simulink model "numerical_lagrangian"  (R2024b)
settings: Solver=ode4  StartTime=0.0  StopTime=8  FixedStep=0.001  RelTol=1e-3
InitFcn:
  | run('assignment_block2.m')
values from neighbouring files (symbols this model uses):
  Acoeffs = computeCoefficients(number_coefficients, tA, tB, qa, qdot_a, qddot_a, qb, qdot_b, qddot_b)    [assignment_block2.m]
  Bcoeffs = computeCoefficients(number_coefficients, tA, tB, qa, qdot_a, qddot_a, qb, qdot_b, qddot_b)    [assignment_block2.m]
  Ccoeffs = computeCoefficients(number_coefficients, tA, tB, qa, qdot_a, qddot_a, qb, qdot_b, qddot_b)    [assignment_block2.m]
  D1 = [1 0 0; 0 0.4 0; 0 0 0.9] .* I0    [assignment_block2.m]
  D2 = [0.45 0 0; 0 1.4 0; 0 0 1.2] .* I0    [assignment_block2.m]
  D3 = D2    [assignment_block2.m]
  D4 = eye(3) .* 0.5 * I0    [assignment_block2.m]
  Dcoeffs = computeCoefficients(number_coefficients, tA, tB, qa, qdot_a, qddot_a, qb, qdot_b, qddot_b)    [assignment_block2.m]
settings Model: Creator=miguelmaidebezares  LastModifiedBy=miguelmaidebezares

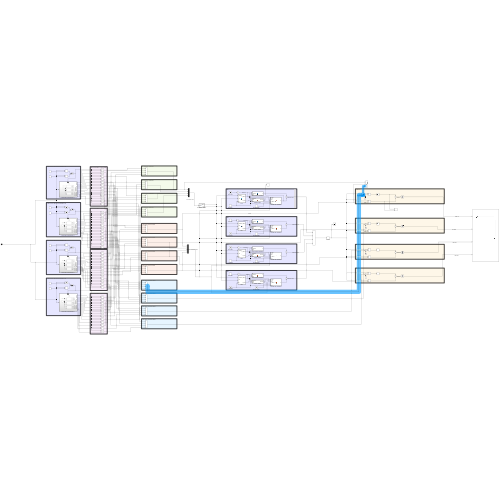
[thumbnail: Simulink's stored preview of the top-level diagram]
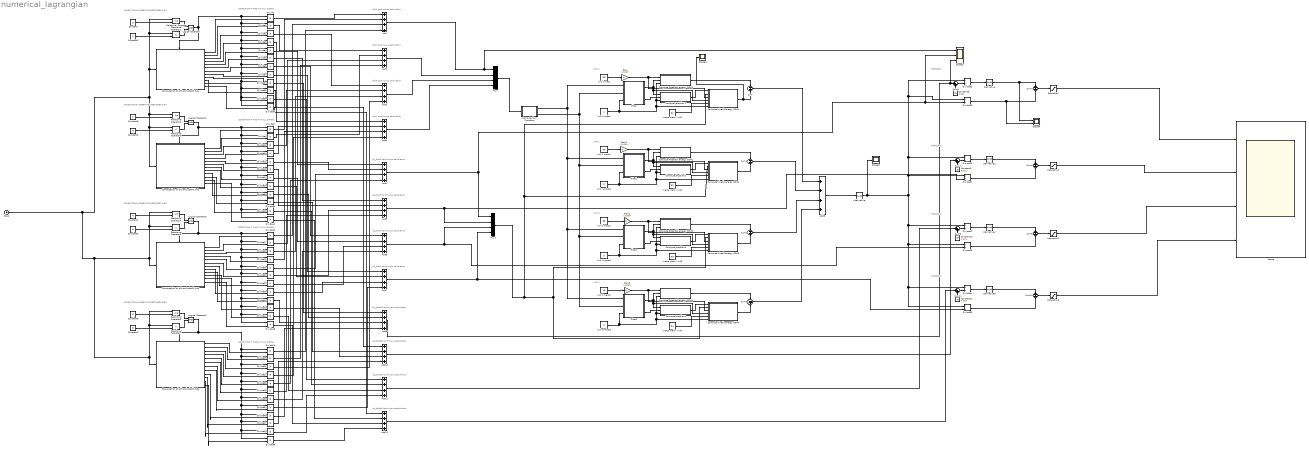
== system numerical_lagrangian ==
  note: TORQUE 1
  note: LINK 1
  note: CONDITION IF AND = 0 KILL SIGNAL
  note: q(t)1 continuous calculation
  note: CONDITIONAL OPERATION BETWEEN 0-2S
  note: CONDITIONAL OPERATION BETWEEN 2-4S
  note: CONDITIONAL OPERATION BETWEEN 4-6S
  note: CONDITIONAL OPERATION BETWEEN 6-8S
  note: CONDITION IF AND = 0 KILL SIGNAL
  note: CONDITION IF AND = 0 KILL SIGNAL
  note: CONDITION IF AND = 0 KILL SIGNAL
  note: q(t)2 continuous calculation
  note: q(t)3 continuous calculation
  note: q(t)4 continuous calculation
  note: q1_dot(t) continuous calculation
  note: q3_dot(t) continuous calculation
  note: q4_dot(t) continuous calculation
  note: q2_dot(t) continuous calculation
  note: LINK 2
  note: LINK 3
  note: LINK 4
  note: q1_ddot(t) continuous calculation
  note: q2_ddot(t) continuous calculation
  note: q3_ddot(t) continuous calculation
  note: q4_ddot(t) continuous calculation
  note: TORQUE 2
  note: TORQUE 2
  note: TORQUE 2
  Add{,1..12} (13 alike) : Sum  Inputs=++++
  Clock : Clock
  Computation of q(t) and qdot(t) 0-2s : Subsystem
  Computation of q(t) and qdot(t) 2-4s : Subsystem
  Computation of q(t) and qdot(t) 4-6s : Subsystem
  Computation of q(t) and qdot(t) 6-8s : Subsystem
  Compute Jacobian 1 : MATLAB Function  TreatAsAtomicUnit=on
  Compute Jacobian2 : MATLAB Function  TreatAsAtomicUnit=on
  Compute Jacobian3 : MATLAB Function  TreatAsAtomicUnit=on
  Compute Jacobian4 : MATLAB Function  TreatAsAtomicUnit=on
  Compute Kinetic energy COM1 : MATLAB Function  TreatAsAtomicUnit=on
  Compute Kinetic energy COM2 : MATLAB Function  TreatAsAtomicUnit=on
  Compute Kinetic energy COM3 : MATLAB Function  TreatAsAtomicUnit=on
  Compute Kinetic energy COM4 : MATLAB Function  TreatAsAtomicUnit=on
  Compute Num Transform : MATLAB Function  TreatAsAtomicUnit=on
  Compute Potential energy COM1 : MATLAB Function  TreatAsAtomicUnit=on
  Compute Potential energy COM2 : MATLAB Function  TreatAsAtomicUnit=on
  Compute Potential energy COM3 : MATLAB Function  TreatAsAtomicUnit=on
  Compute Potential energy COM4 : MATLAB Function  TreatAsAtomicUnit=on
  Constant : Constant  Value=0
  Constant1 : Constant  Value=2
  Constant{8..11} (4 alike) : Constant  Value=0.001
  Constant2 : Constant  Value=2
  Constant3 : Constant  Value=4
  Constant4 : Constant  Value=4
  Constant5 : Constant  Value=6
  Constant6 : Constant  Value=6
  Constant7 : Constant  Value=8
  Derivative{,1..3} (4 alike) : Derivative
  Divide{,1..31,34..49} (48 alike) : Product  Inputs=**
  Divide{32..33,50..55} (8 alike) : Product  Inputs=*/
  Filter : MATLAB Function  TreatAsAtomicUnit=on
  Filter1 : MATLAB Function  TreatAsAtomicUnit=on
  Filter2 : MATLAB Function  TreatAsAtomicUnit=on
  Filter3 : MATLAB Function  TreatAsAtomicUnit=on
  Gain{,1..3} (4 alike) : Gain  Gain=1/1000
  Inertia matrix link1 : Constant  Value=D1
  Inertia matrix link2 : Constant  Value=D2
  Inertia matrix link3 : Constant  Value=D3
  Inertia matrix link4 : Constant  Value=D4
  L derivative : Derivative
  Link 1 mass : Constant  Value=60
  Link 1 mass1 : Constant  Value=80
  Link 1 mass2 : Constant  Value=80
  Link 1 mass3 : Constant  Value=40
  Link number : Constant
  Link number1 : Constant  Value=2
  Link number2 : Constant  Value=3
  Link number3 : Constant  Value=4
  Logical Operator{,1..3} (4 alike) : Logic  AllPortsSameDT=off  OutDataTypeStr=boolean
  Mux : Mux
  Mux1 : Mux
  Relational Operator{,2,4,6} (4 alike) : RelationalOperator  OutDataTypeStr=boolean  RndMeth=Simplest  InputSameDT=off
  Relational Operator{1,3,5,7} (4 alike) : RelationalOperator  Operator=<  OutDataTypeStr=boolean  RndMeth=Simplest  InputSameDT=off
  Saturation{,1..3} (4 alike) : Saturate  UpperLimit=3000  LowerLimit=-2000
  Scope : Scope  NumInputPorts=4
  Scope1 : Scope  NumInputPorts=3
  Scope2 : Scope
  Scope3 : Scope
  Scope4 : Scope  NumInputPorts=2
  Sum{,1..3} (4 alike) : Sum  Inputs=-|+
  Sum{4,6,8,10} (4 alike) : Sum  Inputs=+|-
  Sum{5,7,9,11} (4 alike) : Sum  Inputs=|++
  wires:
  Relational Operator/1 -> Logical Operator/1
  Relational Operator1/1 -> Logical Operator/2
  Constant/1 -> Relational Operator/2
  Constant1/1 -> Relational Operator1/2
  Logical Operator/1 -> Computation of q(t) and qdot(t) 0-2s/Enable, Divide37/1, Divide36/1, Divide35/1, Divide34/1, Divide7/1, Divide6/1, Divide5/1, Divide4/1, Divide3/1, Divide2/1, Divide1/1, Divide/1
  Constant2/1 -> Relational Operator2/2
  Relational Operator3/1 -> Logical Operator1/2
  Constant3/1 -> Relational Operator3/2
  Relational Operator2/1 -> Logical Operator1/1
  Constant4/1 -> Relational Operator4/2
  Relational Operator5/1 -> Logical Operator2/2
  Constant5/1 -> Relational Operator5/2
  Relational Operator4/1 -> Logical Operator2/1
  Constant6/1 -> Relational Operator6/2
  Relational Operator7/1 -> Logical Operator3/2
  Clock/1 -> Computation of q(t) and qdot(t) 2-4s/1(t), Relational Operator3/1, Relational Operator2/1, Relational Operator1/1, Relational Operator/1, Computation of q(t) and qdot(t) 0-2s/1(t), Relational Operator7/1, Relational Operator6/1, Computation of q(t) and qdot(t) 6-8s/1(t), Relational Operator5/1, Relational Operator4/1, Computation of q(t) and qdot(t) 4-6s/1(t)
  Constant7/1 -> Relational Operator7/2
  Relational Operator6/1 -> Logical Operator3/1
  Computation of q(t) and qdot(t) 0-2s/1(q1) -> Divide/2
  Computation of q(t) and qdot(t) 0-2s/2(q2) -> Divide1/2
  Computation of q(t) and qdot(t) 0-2s/3(q3) -> Divide2/2
  Computation of q(t) and qdot(t) 0-2s/4(q4) -> Divide3/2
  Computation of q(t) and qdot(t) 0-2s/5(q1_d) -> Divide4/2
  Computation of q(t) and qdot(t) 0-2s/6(q2_d) -> Divide5/2
  Computation of q(t) and qdot(t) 0-2s/7(q3_d) -> Divide6/2
  Computation of q(t) and qdot(t) 0-2s/8(q4_d) -> Divide7/2
  Divide/1 -> Add/1
  Computation of q(t) and qdot(t) 2-4s/8(q4_d) -> Divide15/2
  Computation of q(t) and qdot(t) 2-4s/2(q2) -> Divide9/2
  Computation of q(t) and qdot(t) 2-4s/6(q2_d) -> Divide13/2
  Computation of q(t) and qdot(t) 2-4s/5(q1_d) -> Divide12/2
  Computation of q(t) and qdot(t) 2-4s/3(q3) -> Divide10/2
  Computation of q(t) and qdot(t) 2-4s/4(q4) -> Divide11/2
  Computation of q(t) and qdot(t) 2-4s/1(q1) -> Divide8/2
  Logical Operator1/1 -> Computation of q(t) and qdot(t) 2-4s/Enable, Divide11/1, Divide41/1, Divide40/1, Divide39/1, Divide38/1, Divide15/1, Divide14/1, Divide13/1, Divide12/1, Divide10/1, Divide9/1, Divide8/1
  Computation of q(t) and qdot(t) 2-4s/7(q3_d) -> Divide14/2
  Computation of q(t) and qdot(t) 4-6s/8(q4_d) -> Divide23/2
  Computation of q(t) and qdot(t) 4-6s/2(q2) -> Divide17/2
  Computation of q(t) and qdot(t) 4-6s/6(q2_d) -> Divide21/2
  Computation of q(t) and qdot(t) 4-6s/5(q1_d) -> Divide20/2
  Computation of q(t) and qdot(t) 4-6s/3(q3) -> Divide18/2
  Computation of q(t) and qdot(t) 4-6s/4(q4) -> Divide19/2
  Computation of q(t) and qdot(t) 4-6s/1(q1) -> Divide16/2
  Computation of q(t) and qdot(t) 4-6s/7(q3_d) -> Divide22/2
  Computation of q(t) and qdot(t) 6-8s/8(q4_d) -> Divide31/2
  Computation of q(t) and qdot(t) 6-8s/2(q2) -> Divide25/2
  Computation of q(t) and qdot(t) 6-8s/6(q2_d) -> Divide29/2
  Computation of q(t) and qdot(t) 6-8s/5(q1_d) -> Divide28/2
  Computation of q(t) and qdot(t) 6-8s/3(q3) -> Divide26/2
  Computation of q(t) and qdot(t) 6-8s/4(q4) -> Divide27/2
  Computation of q(t) and qdot(t) 6-8s/1(q1) -> Divide24/2
  Logical Operator3/1 -> Divide27/1, Divide49/1, Divide48/1, Divide47/1, Divide46/1, Divide31/1, Divide30/1, Divide29/1, Divide28/1, Divide26/1, Divide25/1, Divide24/1, Computation of q(t) and qdot(t) 6-8s/Enable
  Computation of q(t) and qdot(t) 6-8s/7(q3_d) -> Divide30/2
  Divide8/1 -> Add/2
  Divide16/1 -> Add/3
  Divide24/1 -> Add/4
  Divide1/1 -> Add1/1
  Divide9/1 -> Add1/2
  Divide17/1 -> Add1/3
  Divide25/1 -> Add1/4
  Divide2/1 -> Add2/1
  Divide10/1 -> Add2/2
  Divide18/1 -> Add2/3
  Divide26/1 -> Add2/4
  Divide3/1 -> Add3/1
  Divide11/1 -> Add3/2
  Divide19/1 -> Add3/3
  Divide27/1 -> Add3/4
  Divide4/1 -> Add4/1
  Divide12/1 -> Add4/2
  Divide20/1 -> Add4/3
  Divide28/1 -> Add4/4
  Divide5/1 -> Add5/1
  Divide13/1 -> Add5/2
  Divide21/1 -> Add5/3
  Divide29/1 -> Add5/4
  Divide6/1 -> Add6/1
  Divide14/1 -> Add6/2
  Divide22/1 -> Add6/3
  Divide30/1 -> Add6/4
  Divide7/1 -> Add7/1
  Divide15/1 -> Add7/2
  Divide23/1 -> Add7/3
  Divide31/1 -> Add7/4
  Add1/1 -> Mux/2
  Add2/1 -> Mux/3
  Add3/1 -> Mux/4
  Mux/1 -> Compute Num Transform/1(poses)  "poses (q1, q2, q3, q4)"
  Add4/1 -> Scope1/2, Divide33/2, Mux1/1  "Q1 DOT"
  Link number/1 -> Compute Kinetic energy COM1/6(link_n), Compute Jacobian 1/3(link_n), Compute Potential energy COM1/3(link_n), Filter/3(link_n)
  Filter/1(T_COMcell) -> Compute Kinetic energy COM1/4(T_COMlist), Compute Jacobian 1/1(T_COMlist), Compute Potential energy COM1/2(T_COMlist)
  Filter/2(T_listcell) -> Compute Jacobian 1/2(T_list)
  Link 1 mass/1 -> Gain/1
  Compute Jacobian 1/1(jacobian) -> Compute Kinetic energy COM1/1(jacobian)
  Inertia matrix link1/1 -> Compute Kinetic energy COM1/5(I)
  Compute Potential energy COM1/1(P) -> Sum/1
  Compute Kinetic energy COM1/1(K) -> Scope2/1, Sum/2
  Sum/1 -> Add8/1  "Lagrangian comp L1"
  Filter1/2(T_listcell) -> Compute Jacobian2/2(T_list)
  Compute Jacobian2/1(jacobian) -> Compute Kinetic energy COM2/1(jacobian)
  Filter1/1(T_COMcell) -> Compute Kinetic energy COM2/4(T_COMlist), Compute Jacobian2/1(T_COMlist), Compute Potential energy COM2/2(T_COMlist)
  Link number1/1 -> Compute Kinetic energy COM2/6(link_n), Compute Jacobian2/3(link_n), Compute Potential energy COM2/3(link_n), Filter1/3(link_n)
  Inertia matrix link2/1 -> Compute Kinetic energy COM2/5(I)
  Mux1/1 -> Compute Kinetic energy COM2/2(q_dot), Compute Kinetic energy COM1/2(q_dot), Compute Kinetic energy COM4/2(q_dot), Compute Kinetic energy COM3/2(q_dot)  "poses (qdot1, qdot2, qdot3, qdot4)"
  Compute Potential energy COM2/1(P) -> Sum1/1
  Link 1 mass1/1 -> Gain1/1
  Compute Kinetic energy COM2/1(K) -> Sum1/2
  Sum1/1 -> Add8/2  "Lagrangian comp L2"
  Filter2/2(T_listcell) -> Compute Jacobian3/2(T_list)
  Compute Jacobian3/1(jacobian) -> Compute Kinetic energy COM3/1(jacobian)
  Filter2/1(T_COMcell) -> Compute Kinetic energy COM3/4(T_COMlist), Compute Jacobian3/1(T_COMlist), Compute Potential energy COM3/2(T_COMlist)
  Link number2/1 -> Compute Kinetic energy COM3/6(link_n), Compute Jacobian3/3(link_n), Compute Potential energy COM3/3(link_n), Filter2/3(link_n)
  Inertia matrix link3/1 -> Compute Kinetic energy COM3/5(I)
  Compute Potential energy COM3/1(P) -> Sum2/1
  Link 1 mass2/1 -> Gain2/1
  Compute Kinetic energy COM3/1(K) -> Sum2/2
  Sum2/1 -> Add8/3  "Lagrangian comp L3"
  Compute Num Transform/1(T_COMlist) -> Filter/1(T_COMlist), Filter3/1(T_COMlist), Filter2/1(T_COMlist), Filter1/1(T_COMlist)
  Filter3/2(T_listcell) -> Compute Jacobian4/2(T_list)
  Compute Jacobian4/1(jacobian) -> Compute Kinetic energy COM4/1(jacobian)
  Filter3/1(T_COMcell) -> Compute Kinetic energy COM4/4(T_COMlist), Compute Jacobian4/1(T_COMlist), Compute Potential energy COM4/2(T_COMlist)
  Link number3/1 -> Compute Kinetic energy COM4/6(link_n), Compute Jacobian4/3(link_n), Compute Potential energy COM4/3(link_n), Filter3/3(link_n)
  Inertia matrix link4/1 -> Compute Kinetic energy COM4/5(I)
  Compute Num Transform/2(T_list) -> Filter3/2(T_list), Filter2/2(T_list), Filter1/2(T_list), Filter/2(T_list)
  Compute Potential energy COM4/1(P) -> Sum3/1
  Link 1 mass3/1 -> Gain3/1
  Compute Kinetic energy COM4/1(K) -> Sum3/2
  Sum3/1 -> Add8/4  "Lagrangian comp L4"
  Add8/1 -> L derivative/1
  Divide32/1 -> Derivative/1
  Divide33/1 -> Scope4/2, Sum4/2
  Sum4/1 -> Saturation/1  "TORQUE1"
  Gain/1 -> Compute Kinetic energy COM1/3(mass), Compute Potential energy COM1/1(m)  "mass in kg"
  Gain1/1 -> Compute Kinetic energy COM2/3(mass), Compute Potential energy COM2/1(m)  "mass in kg"
  Gain2/1 -> Compute Kinetic energy COM3/3(mass), Compute Potential energy COM3/1(m)  "mass in kg"
  Gain3/1 -> Compute Kinetic energy COM4/3(mass), Compute Potential energy COM4/1(m)  "mass in kg"
  Add/1 -> Scope1/1, Mux/1
  Computation of q(t) and qdot(t) 0-2s/9(q1_dd) -> Divide34/2
  Computation of q(t) and qdot(t) 0-2s/10(q2_dd) -> Divide35/2
  Computation of q(t) and qdot(t) 0-2s/11(q3_dd) -> Divide36/2
  Computation of q(t) and qdot(t) 0-2s/12(q4_dd) -> Divide37/2
  Computation of q(t) and qdot(t) 2-4s/9(q1_dd) -> Divide38/2
  Computation of q(t) and qdot(t) 2-4s/10(q2_dd) -> Divide39/2
  Computation of q(t) and qdot(t) 2-4s/11(q3_dd) -> Divide40/2
  Computation of q(t) and qdot(t) 2-4s/12(q4_dd) -> Divide41/2
  Computation of q(t) and qdot(t) 4-6s/9(q1_dd) -> Divide42/2
  Computation of q(t) and qdot(t) 4-6s/10(q2_dd) -> Divide43/2
  Computation of q(t) and qdot(t) 4-6s/11(q3_dd) -> Divide44/2
  Computation of q(t) and qdot(t) 4-6s/12(q4_dd) -> Divide45/2
  Logical Operator2/1 -> Divide19/1, Divide45/1, Divide44/1, Divide43/1, Divide42/1, Divide23/1, Divide22/1, Divide21/1, Divide20/1, Divide18/1, Divide17/1, Divide16/1, Computation of q(t) and qdot(t) 4-6s/Enable
  Computation of q(t) and qdot(t) 6-8s/9(q1_dd) -> Divide46/2
  Computation of q(t) and qdot(t) 6-8s/10(q2_dd) -> Divide47/2
  Computation of q(t) and qdot(t) 6-8s/11(q3_dd) -> Divide48/2
  Computation of q(t) and qdot(t) 6-8s/12(q4_dd) -> Divide49/2
  Divide34/1 -> Add9/1
  Divide35/1 -> Add10/1
  Divide42/1 -> Add9/3
  Divide46/1 -> Add9/4
  Divide36/1 -> Add11/1
  Divide37/1 -> Add12/1
  Divide38/1 -> Add9/2
  Divide39/1 -> Add10/2
  Divide40/1 -> Add11/2
  Divide41/1 -> Add12/2
  Divide43/1 -> Add10/3
  Divide44/1 -> Add11/3
  Divide47/1 -> Add10/4
  Divide48/1 -> Add11/4
  Divide49/1 -> Add12/4
  Divide45/1 -> Add12/3
  Add9/1 -> Sum5/1, Scope1/3  "Q1  DOUBLE DOT"
  Constant8/1 -> Sum5/2
  Sum5/1 -> Divide32/2
  Derivative/1 -> Scope4/1, Sum4/1
  Saturation/1 -> Scope/1  "TORQUE1"
  Sum6/1 -> Saturation1/1  "TORQUE2"
  Derivative1/1 -> Sum6/1
  Divide51/1 -> Sum6/2
  Divide50/1 -> Derivative1/1
  Saturation1/1 -> Scope/2  "TORQUE2"
  Add5/1 -> Divide51/2, Mux1/2  "Q2 DOT"
  Add10/1 -> Sum7/1
  Constant9/1 -> Sum7/2
  Sum7/1 -> Divide50/2
  Divide53/1 -> Sum8/2
  Add6/1 -> Divide53/2, Mux1/3
  Constant10/1 -> Sum9/2
  Derivative2/1 -> Sum8/1
  Saturation2/1 -> Scope/3  "TORQUE3"
  Sum8/1 -> Saturation2/1  "TORQUE2"
  Sum9/1 -> Divide52/2
  Divide52/1 -> Derivative2/1
  Divide55/1 -> Sum10/2
  L derivative/1 -> Divide51/1, Divide33/1, Divide32/1, Divide50/1, Divide53/1, Divide55/1, Divide54/1, Divide52/1, Scope3/1
  Constant11/1 -> Sum11/2
  Derivative3/1 -> Sum10/1
  Saturation3/1 -> Scope/4  "TORQUE4"
  Sum10/1 -> Saturation3/1  "TORQUE2"
  Sum11/1 -> Divide54/2
  Add12/1 -> Sum11/1
  Divide54/1 -> Derivative3/1
  Add7/1 -> Divide55/2, Mux1/4
  Add11/1 -> Sum9/1

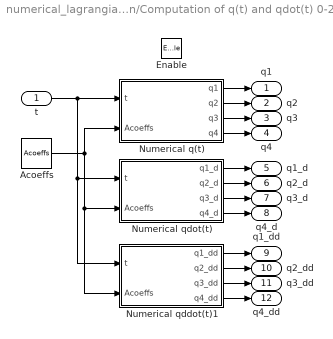
== system numerical_lagrangian/Computation of q(t) and qdot(t) 0-2s ==
  t : Inport
  Enable : EnablePort
  Acoeffs : Constant  Value=Acoeffs
  Numerical q(t) : MATLAB Function  TreatAsAtomicUnit=on
  Numerical qddot(t)1 : MATLAB Function  TreatAsAtomicUnit=on
  Numerical qdot(t) : MATLAB Function  TreatAsAtomicUnit=on
  q1 : Outport  OutDataTypeStr=double
  q2 : Outport  Port=2
  q3 : Outport  Port=3
  q4 : Outport  Port=4
  q1_d : Outport  Port=5
  q2_d : Outport  Port=6
  q3_d : Outport  Port=7
  q4_d : Outport  Port=8
  q1_dd : Outport  Port=9
  q2_dd : Outport  Port=10
  q3_dd : Outport  Port=11
  q4_dd : Outport  Port=12
  wires:
  Numerical q(t)/3(q3) -> q3/1
  Numerical qdot(t)/3(q3_d) -> q3_d/1
  Numerical q(t)/2(q2) -> q2/1
  Numerical q(t)/1(q1) -> q1/1
  Numerical qdot(t)/2(q2_d) -> q2_d/1
  Numerical qdot(t)/4(q4_d) -> q4_d/1
  Numerical q(t)/4(q4) -> q4/1
  Numerical qdot(t)/1(q1_d) -> q1_d/1
  Acoeffs/1 -> Numerical q(t)/2(Acoeffs), Numerical qddot(t)1/2(Acoeffs), Numerical qdot(t)/2(Acoeffs)
  t/1 -> Numerical qddot(t)1/1(t), Numerical qdot(t)/1(t), Numerical q(t)/1(t)
  Numerical qddot(t)1/1(q1_dd) -> q1_dd/1
  Numerical qddot(t)1/2(q2_dd) -> q2_dd/1
  Numerical qddot(t)1/3(q3_dd) -> q3_dd/1
  Numerical qddot(t)1/4(q4_dd) -> q4_dd/1

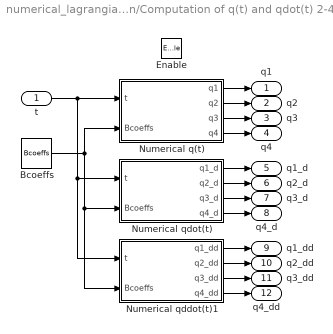
== system numerical_lagrangian/Computation of q(t) and qdot(t) 2-4s ==
  t : Inport
  Enable : EnablePort
  Bcoeffs : Constant  Value=Bcoeffs
  Numerical q(t) : MATLAB Function  TreatAsAtomicUnit=on
  Numerical qddot(t)1 : MATLAB Function  TreatAsAtomicUnit=on
  Numerical qdot(t) : MATLAB Function  TreatAsAtomicUnit=on
  q1 : Outport  OutDataTypeStr=double
  q2 : Outport  Port=2
  q3 : Outport  Port=3
  q4 : Outport  Port=4
  q1_d : Outport  Port=5
  q2_d : Outport  Port=6
  q3_d : Outport  Port=7
  q4_d : Outport  Port=8
  q1_dd : Outport  Port=9
  q2_dd : Outport  Port=10
  q3_dd : Outport  Port=11
  q4_dd : Outport  Port=12
  wires:
  Numerical q(t)/3(q3) -> q3/1
  Numerical qdot(t)/3(q3_d) -> q3_d/1
  Numerical q(t)/2(q2) -> q2/1
  Numerical q(t)/1(q1) -> q1/1
  Numerical qdot(t)/2(q2_d) -> q2_d/1
  Numerical qdot(t)/4(q4_d) -> q4_d/1
  Numerical q(t)/4(q4) -> q4/1
  Numerical qdot(t)/1(q1_d) -> q1_d/1
  Numerical qddot(t)1/2(q2_dd) -> q2_dd/1
  Bcoeffs/1 -> Numerical q(t)/2(Bcoeffs), Numerical qddot(t)1/2(Bcoeffs), Numerical qdot(t)/2(Bcoeffs)
  Numerical qddot(t)1/1(q1_dd) -> q1_dd/1
  t/1 -> Numerical qddot(t)1/1(t), Numerical qdot(t)/1(t), Numerical q(t)/1(t)
  Numerical qddot(t)1/3(q3_dd) -> q3_dd/1
  Numerical qddot(t)1/4(q4_dd) -> q4_dd/1

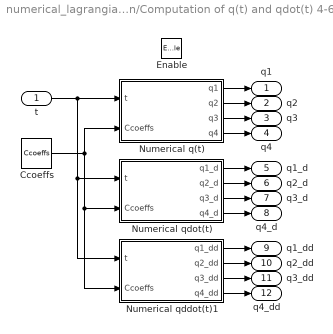
== system numerical_lagrangian/Computation of q(t) and qdot(t) 4-6s ==
  t : Inport
  Enable : EnablePort
  Ccoeffs : Constant  Value=Ccoeffs
  Numerical q(t) : MATLAB Function  TreatAsAtomicUnit=on
  Numerical qddot(t)1 : MATLAB Function  TreatAsAtomicUnit=on
  Numerical qdot(t) : MATLAB Function  TreatAsAtomicUnit=on
  q1 : Outport  OutDataTypeStr=double
  q2 : Outport  Port=2
  q3 : Outport  Port=3
  q4 : Outport  Port=4
  q1_d : Outport  Port=5
  q2_d : Outport  Port=6
  q3_d : Outport  Port=7
  q4_d : Outport  Port=8
  q1_dd : Outport  Port=9
  q2_dd : Outport  Port=10
  q3_dd : Outport  Port=11
  q4_dd : Outport  Port=12
  wires:
  Numerical q(t)/3(q3) -> q3/1
  Numerical qdot(t)/3(q3_d) -> q3_d/1
  Numerical q(t)/2(q2) -> q2/1
  Numerical q(t)/1(q1) -> q1/1
  Numerical qdot(t)/2(q2_d) -> q2_d/1
  Numerical qdot(t)/4(q4_d) -> q4_d/1
  Numerical q(t)/4(q4) -> q4/1
  Numerical qdot(t)/1(q1_d) -> q1_d/1
  Numerical qddot(t)1/2(q2_dd) -> q2_dd/1
  Ccoeffs/1 -> Numerical q(t)/2(Ccoeffs), Numerical qddot(t)1/2(Ccoeffs), Numerical qdot(t)/2(Ccoeffs)
  Numerical qddot(t)1/1(q1_dd) -> q1_dd/1
  t/1 -> Numerical qddot(t)1/1(t), Numerical qdot(t)/1(t), Numerical q(t)/1(t)
  Numerical qddot(t)1/3(q3_dd) -> q3_dd/1
  Numerical qddot(t)1/4(q4_dd) -> q4_dd/1

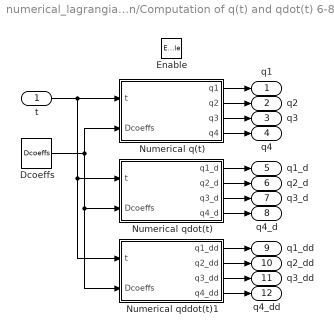
== system numerical_lagrangian/Computation of q(t) and qdot(t) 6-8s ==
  t : Inport
  Enable : EnablePort
  Dcoeffs : Constant  Value=Dcoeffs
  Numerical q(t) : MATLAB Function  TreatAsAtomicUnit=on
  Numerical qddot(t)1 : MATLAB Function  TreatAsAtomicUnit=on
  Numerical qdot(t) : MATLAB Function  TreatAsAtomicUnit=on
  q1 : Outport  OutDataTypeStr=double
  q2 : Outport  Port=2
  q3 : Outport  Port=3
  q4 : Outport  Port=4
  q1_d : Outport  Port=5
  q2_d : Outport  Port=6
  q3_d : Outport  Port=7
  q4_d : Outport  Port=8
  q1_dd : Outport  Port=9
  q2_dd : Outport  Port=10
  q3_dd : Outport  Port=11
  q4_dd : Outport  Port=12
  wires:
  Numerical q(t)/3(q3) -> q3/1
  Numerical qdot(t)/3(q3_d) -> q3_d/1
  Numerical q(t)/2(q2) -> q2/1
  Numerical q(t)/1(q1) -> q1/1
  Numerical qdot(t)/2(q2_d) -> q2_d/1
  Numerical qdot(t)/4(q4_d) -> q4_d/1
  Numerical q(t)/4(q4) -> q4/1
  Numerical qdot(t)/1(q1_d) -> q1_d/1
  Numerical qddot(t)1/2(q2_dd) -> q2_dd/1
  Dcoeffs/1 -> Numerical q(t)/2(Dcoeffs), Numerical qddot(t)1/2(Dcoeffs), Numerical qdot(t)/2(Dcoeffs)
  Numerical qddot(t)1/1(q1_dd) -> q1_dd/1
  t/1 -> Numerical qddot(t)1/1(t), Numerical qdot(t)/1(t), Numerical q(t)/1(t)
  Numerical qddot(t)1/3(q3_dd) -> q3_dd/1
  Numerical qddot(t)1/4(q4_dd) -> q4_dd/1

== matlab function numerical_lagrangian/Compute Num Transform ==
  data: poses input; T_COMlist output; T_list output
function [T_COMlist, T_list] = fcn(poses)

    [T_COMlist, T_list] = computeNumericTransform(poses);

end

== matlab function numerical_lagrangian/Compute Jacobian 1 ==
  data: T_COMlist input; jacobian output size=[6 4]; T_list input; link_n input
function jacobian = fcn(T_COMlist, T_list, link_n)
%#codegen
    jacobian = computeJacobianCOM(T_COMlist, T_list, link_n);
end

== matlab function numerical_lagrangian/Filter ==
  data: T_COMcell output size=[4 4 4]; T_COMlist input; T_list input; T_listcell output size=[4 4 4]; link_n input
function [T_COMcell, T_listcell] = fcn(T_COMlist, T_list, link_n)
%#codegen

    % We know there are at most 4 links.
    % Always output 4x4x4 (fixed size) for Simulink.

    T_COMcell  = zeros(4,4,4);
    T_listcell = zeros(4,4,4);

    for k = 1:4
        if k <= link_n
            T_COMcell(:,:,k)  = T_COMlist(:,:,k);
            T_listcell(:,:,k) = T_list(:,:,k);
        else
            % You can leave as zeros, or use eye(4) if that’s more meaningful:
            % T_COMcell(:,:,k)  = eye(4);
            % T_listcell(:,:,k) = eye(4);
        end
    end
end

== matlab function numerical_lagrangian/Computation of q(t) and qdot(t) 0-2s/Numerical qdot(t) ==
  data: t input; Acoeffs input; q1_d output; q2_d output; q3_d output; q4_d output
function [q1_d, q2_d, q3_d, q4_d] = fcn(t, Acoeffs)
    
    d1 = polyder(Acoeffs(1, :));
    d2 = polyder(Acoeffs(2, :));
    d3 = polyder(Acoeffs(3, :));
    d4 = polyder(Acoeffs(4, :));

    q1_d = sum(computeNumVect(d1, t));
    q2_d = sum(computeNumVect(d2, t));
    q3_d = sum(computeNumVect(d3, t));
    q4_d = sum(computeNumVect(d4, t));
end

== matlab function numerical_lagrangian/Compute Potential energy COM1 ==
  data: m input; P output; T_COMlist input; link_n input
function P = fcn(m, T_COMlist, link_n)
    % Compute the potential energy of the COM of the first link
    T_COM = T_COMlist(:, :, link_n);
    COM_z = T_COM(3, 4);
    P = computeP(m, COM_z);
end

== matlab function numerical_lagrangian/Compute Kinetic energy COM1 ==
  data: jacobian input; K output; q_dot input; mass input; T_COMlist input; I input; link_n input
function K = fcn(jacobian, q_dot, mass, T_COMlist, I, link_n)

    % TCOM_list wrapper here

    T = T_COMlist(:, :, link_n);

    K = computeK(jacobian, q_dot, mass, T, I);

end

== matlab function numerical_lagrangian/Compute Jacobian2 ==
  data: T_COMlist input; jacobian output size=[6 4]; T_list input; link_n input
function jacobian = fcn(T_COMlist, T_list, link_n)

    jacobian = computeJacobianCOM(T_COMlist, T_list, link_n);

end

== matlab function numerical_lagrangian/Compute Kinetic energy COM2 ==
  data: jacobian input; K output; q_dot input; mass input; T_COMlist input; I input; link_n input
function K = fcn(jacobian, q_dot, mass, T_COMlist, I, link_n)

    % TCOM_list wrapper here

    T = T_COMlist(:, :, link_n);

    K = computeK(jacobian, q_dot, mass, T, I);

end

== matlab function numerical_lagrangian/Compute Potential energy COM2 ==
  data: m input; P output; T_COMlist input; link_n input
function P = fcn(m, T_COMlist, link_n)
    % Compute the potential energy of the COM of the second link
    T_COM = T_COMlist(:, :, link_n);
    COM_z = T_COM(3, 4);
    P = computeP(m, COM_z);
end

== matlab function numerical_lagrangian/Filter1 ==
  data: T_COMcell output size=[4 4 4]; T_COMlist input; T_list input; T_listcell output size=[4 4 4]; link_n input
function [T_COMcell, T_listcell] = fcn(T_COMlist, T_list, link_n)
%#codegen

    % We know there are at most 4 links.
    % Always output 4x4x4 (fixed size) for Simulink.

    T_COMcell  = zeros(4,4,4);
    T_listcell = zeros(4,4,4);

    for k = 1:4
        if k <= link_n
            T_COMcell(:,:,k)  = T_COMlist(:,:,k);
            T_listcell(:,:,k) = T_list(:,:,k);
        else
            % You can leave as zeros, or use eye(4) if that’s more meaningful:
            % T_COMcell(:,:,k)  = eye(4);
            % T_listcell(:,:,k) = eye(4);
        end
    end
end

== matlab function numerical_lagrangian/Compute Jacobian3 ==
  data: T_COMlist input; jacobian output size=[6 4]; T_list input; link_n input
function jacobian = fcn(T_COMlist, T_list, link_n)

    jacobian = computeJacobianCOM(T_COMlist, T_list, link_n);

end

== matlab function numerical_lagrangian/Compute Kinetic energy COM3 ==
  data: jacobian input; K output; q_dot input; mass input; T_COMlist input; I input; link_n input
function K = fcn(jacobian, q_dot, mass, T_COMlist, I, link_n)

    % TCOM_list wrapper here

    T = T_COMlist(:, :, link_n);

    K = computeK(jacobian, q_dot, mass, T, I);

end

== matlab function numerical_lagrangian/Compute Potential energy COM3 ==
  data: m input; P output; T_COMlist input; link_n input
function P = fcn(m, T_COMlist, link_n)
    % Compute the potential energy of the COM of the first link
    T_COM = T_COMlist(:, :, link_n);
    COM_z = T_COM(3, 4);
    P = computeP(m, COM_z);
end

== matlab function numerical_lagrangian/Filter2 ==
  data: T_COMcell output size=[4 4 4]; T_COMlist input; T_list input; T_listcell output size=[4 4 4]; link_n input
function [T_COMcell, T_listcell] = fcn(T_COMlist, T_list, link_n)
%#codegen

    % We know there are at most 4 links.
    % Always output 4x4x4 (fixed size) for Simulink.

    T_COMcell  = zeros(4,4,4);
    T_listcell = zeros(4,4,4);

    for k = 1:4
        if k <= link_n
            T_COMcell(:,:,k)  = T_COMlist(:,:,k);
            T_listcell(:,:,k) = T_list(:,:,k);
        else
            % You can leave as zeros, or use eye(4) if that’s more meaningful:
            % T_COMcell(:,:,k)  = eye(4);
            % T_listcell(:,:,k) = eye(4);
        end
    end
end

== matlab function numerical_lagrangian/Compute Jacobian4 ==
  data: T_COMlist input; jacobian output size=[6 4]; T_list input; link_n input
function jacobian = fcn(T_COMlist, T_list, link_n)

    jacobian = computeJacobianCOM(T_COMlist, T_list, link_n);

end

== matlab function numerical_lagrangian/Computation of q(t) and qdot(t) 0-2s/Numerical q(t) ==
  data: t input; q1 output; q2 output; q3 output; q4 output; Acoeffs input
function [q1, q2, q3, q4] = fcn(t, Acoeffs)

    q1 = sum(computeNumVect(Acoeffs(1, :), t));
    q2 = sum(computeNumVect(Acoeffs(2, :), t));
    q3 = sum(computeNumVect(Acoeffs(3, :), t));
    q4 = sum(computeNumVect(Acoeffs(4, :), t));

end

== matlab function numerical_lagrangian/Compute Kinetic energy COM4 ==
  data: jacobian input; K output; q_dot input; mass input; T_COMlist input; I input; link_n input
function K = fcn(jacobian, q_dot, mass, T_COMlist, I, link_n)

    % TCOM_list wrapper here

    T = T_COMlist(:, :, link_n);

    K = computeK(jacobian, q_dot, mass, T, I);

end

== matlab function numerical_lagrangian/Compute Potential energy COM4 ==
  data: m input; P output; T_COMlist input; link_n input
function P = fcn(m, T_COMlist, link_n)
    % Compute the potential energy of the COM of the first link
    T_COM = T_COMlist(:, :, link_n);
    COM_z = T_COM(3, 4);
    P = computeP(m, COM_z);
end

== matlab function numerical_lagrangian/Filter3 ==
  data: T_COMcell output size=[4 4 4]; T_COMlist input; T_list input; T_listcell output size=[4 4 4]; link_n input
function [T_COMcell, T_listcell] = fcn(T_COMlist, T_list, link_n)
%#codegen

    % We know there are at most 4 links.
    % Always output 4x4x4 (fixed size) for Simulink.

    T_COMcell  = zeros(4,4,4);
    T_listcell = zeros(4,4,4);

    for k = 1:4
        if k <= link_n
            T_COMcell(:,:,k)  = T_COMlist(:,:,k);
            T_listcell(:,:,k) = T_list(:,:,k);
        else
            % You can leave as zeros, or use eye(4) if that’s more meaningful:
            % T_COMcell(:,:,k)  = eye(4);
            % T_listcell(:,:,k) = eye(4);
        end
    end
end

== matlab function numerical_lagrangian/Computation of q(t) and qdot(t) 0-2s/Numerical qddot(t)1 ==
  data: t input; Acoeffs input; q1_dd output; q2_dd output; q3_dd output; q4_dd output
function [q1_dd, q2_dd, q3_dd, q4_dd] = fcn(t, Acoeffs)
    
    d1 = polyder(polyder(Acoeffs(1, :)));
    d2 = polyder(polyder(Acoeffs(2, :)));
    d3 = polyder(polyder(Acoeffs(3, :)));
    d4 = polyder(polyder(Acoeffs(4, :)));

    q1_dd = sum(computeNumVect(d1, t));
    q2_dd = sum(computeNumVect(d2, t));
    q3_dd = sum(computeNumVect(d3, t));
    q4_dd = sum(computeNumVect(d4, t));
end

== matlab function numerical_lagrangian/Computation of q(t) and qdot(t) 2-4s/Numerical qddot(t)1 ==
  data: t input; Bcoeffs input; q1_dd output; q2_dd output; q3_dd output; q4_dd output
function [q1_dd, q2_dd, q3_dd, q4_dd] = fcn(t, Bcoeffs)
    
    d1 = polyder(polyder(Bcoeffs(1, :)));
    d2 = polyder(polyder(Bcoeffs(2, :)));
    d3 = polyder(polyder(Bcoeffs(3, :)));
    d4 = polyder(polyder(Bcoeffs(4, :)));

    q1_dd = sum(computeNumVect(d1, t));
    q2_dd = sum(computeNumVect(d2, t));
    q3_dd = sum(computeNumVect(d3, t));
    q4_dd = sum(computeNumVect(d4, t));
end

== matlab function numerical_lagrangian/Computation of q(t) and qdot(t) 4-6s/Numerical qddot(t)1 ==
  data: t input; Ccoeffs input; q1_dd output; q2_dd output; q3_dd output; q4_dd output
function [q1_dd, q2_dd, q3_dd, q4_dd] = fcn(t, Ccoeffs)
    
    d1 = polyder(polyder(Ccoeffs(1, :)));
    d2 = polyder(polyder(Ccoeffs(2, :)));
    d3 = polyder(polyder(Ccoeffs(3, :)));
    d4 = polyder(polyder(Ccoeffs(4, :)));

    q1_dd = sum(computeNumVect(d1, t));
    q2_dd = sum(computeNumVect(d2, t));
    q3_dd = sum(computeNumVect(d3, t));
    q4_dd = sum(computeNumVect(d4, t));
end

== matlab function numerical_lagrangian/Computation of q(t) and qdot(t) 6-8s/Numerical qddot(t)1 ==
  data: t input; Dcoeffs input; q1_dd output; q2_dd output; q3_dd output; q4_dd output
function [q1_dd, q2_dd, q3_dd, q4_dd] = fcn(t, Dcoeffs)
    
    d1 = polyder(polyder(Dcoeffs(1, :)));
    d2 = polyder(polyder(Dcoeffs(2, :)));
    d3 = polyder(polyder(Dcoeffs(3, :)));
    d4 = polyder(polyder(Dcoeffs(4, :)));

    q1_dd = sum(computeNumVect(d1, t));
    q2_dd = sum(computeNumVect(d2, t));
    q3_dd = sum(computeNumVect(d3, t));
    q4_dd = sum(computeNumVect(d4, t));
end

== matlab function numerical_lagrangian/Computation of q(t) and qdot(t) 2-4s/Numerical q(t) ==
  data: t input; q1 output; q2 output; q3 output; q4 output; Bcoeffs input
function [q1, q2, q3, q4] = fcn(t, Bcoeffs)

    q1 = sum(computeNumVect(Bcoeffs(1, :), t));
    q2 = sum(computeNumVect(Bcoeffs(2, :), t));
    q3 = sum(computeNumVect(Bcoeffs(3, :), t));
    q4 = sum(computeNumVect(Bcoeffs(4, :), t));

end

== matlab function numerical_lagrangian/Computation of q(t) and qdot(t) 2-4s/Numerical qdot(t) ==
  data: t input; Bcoeffs input; q1_d output; q2_d output; q3_d output; q4_d output
function [q1_d, q2_d, q3_d, q4_d] = fcn(t, Bcoeffs)
    
    d1 = polyder(Bcoeffs(1, :));
    d2 = polyder(Bcoeffs(2, :));
    d3 = polyder(Bcoeffs(3, :));
    d4 = polyder(Bcoeffs(4, :));

    q1_d = sum(computeNumVect(d1, t));
    q2_d = sum(computeNumVect(d2, t));
    q3_d = sum(computeNumVect(d3, t));
    q4_d = sum(computeNumVect(d4, t));
end

== matlab function numerical_lagrangian/Computation of q(t) and qdot(t) 4-6s/Numerical q(t) ==
  data: t input; q1 output; q2 output; q3 output; q4 output; Ccoeffs input
function [q1, q2, q3, q4] = fcn(t, Ccoeffs)

    q1 = sum(computeNumVect(Ccoeffs(1, :), t));
    q2 = sum(computeNumVect(Ccoeffs(2, :), t));
    q3 = sum(computeNumVect(Ccoeffs(3, :), t));
    q4 = sum(computeNumVect(Ccoeffs(4, :), t));

end

== matlab function numerical_lagrangian/Computation of q(t) and qdot(t) 4-6s/Numerical qdot(t) ==
  data: t input; Ccoeffs input; q1_d output; q2_d output; q3_d output; q4_d output
function [q1_d, q2_d, q3_d, q4_d] = fcn(t, Ccoeffs)
    
    d1 = polyder(Ccoeffs(1, :));
    d2 = polyder(Ccoeffs(2, :));
    d3 = polyder(Ccoeffs(3, :));
    d4 = polyder(Ccoeffs(4, :));

    q1_d = sum(computeNumVect(d1, t));
    q2_d = sum(computeNumVect(d2, t));
    q3_d = sum(computeNumVect(d3, t));
    q4_d = sum(computeNumVect(d4, t));
end

== matlab function numerical_lagrangian/Computation of q(t) and qdot(t) 6-8s/Numerical q(t) ==
  data: t input; q1 output; q2 output; q3 output; q4 output; Dcoeffs input
function [q1, q2, q3, q4] = fcn(t, Dcoeffs)

    q1 = sum(computeNumVect(Dcoeffs(1, :), t));
    q2 = sum(computeNumVect(Dcoeffs(2, :), t));
    q3 = sum(computeNumVect(Dcoeffs(3, :), t));
    q4 = sum(computeNumVect(Dcoeffs(4, :), t));

end

== matlab function numerical_lagrangian/Computation of q(t) and qdot(t) 6-8s/Numerical qdot(t) ==
  data: t input; Dcoeffs input; q1_d output; q2_d output; q3_d output; q4_d output
function [q1_d, q2_d, q3_d, q4_d] = fcn(t, Dcoeffs)
    
    d1 = polyder(Dcoeffs(1, :));
    d2 = polyder(Dcoeffs(2, :));
    d3 = polyder(Dcoeffs(3, :));
    d4 = polyder(Dcoeffs(4, :));

    q1_d = sum(computeNumVect(d1, t));
    q2_d = sum(computeNumVect(d2, t));
    q3_d = sum(computeNumVect(d3, t));
    q4_d = sum(computeNumVect(d4, t));
end
